simulink model "myhydro2pumps_iov1"  (Simulink 7.4)
settings: Solver=ode1  StartTime=0.0  StopTime=inf  FixedStep=0.5  RelTol=1e-3  AbsTol=1e-6
undefined symbols (not defined in the file or in its folder): calibParams, Q1max
libraries: hydro2pumps_lib x1
settings Model: Creator=dmedonza  LastModifiedBy=student
settings DataIOCC: LimitDataPoints=off  SignalLoggingName=sigsOut
settings OptimizationCC: BooleanDataType=off
settings DebuggingCC: SaveWithParameterizedLinksMsg=none  SignalResolutionControl=TryResolveAllWithWarning  SolverPrmCheckMsg=none  MultiTaskDSMMsg=warning  MultiTaskCondExecSysMsg=none  StrictBusMsg=None
settings HardwareCC: TargetUnknown=on
settings RTWCC: TemplateMakefile=grt_vc.tmf  IncludeERTFirstTime=on

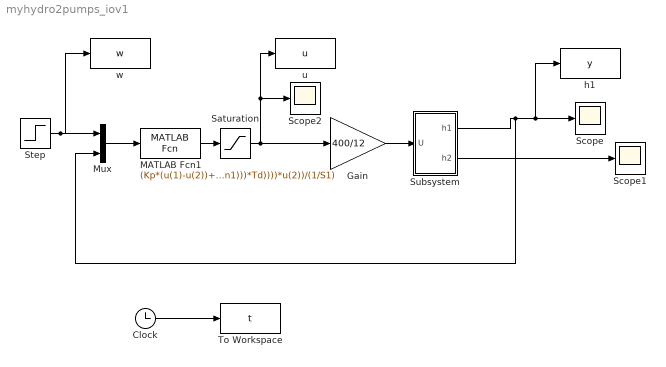
== system myhydro2pumps_iov1 ==
  Clock : Clock
      settings: Decimation=10
  Gain : Gain  Gain=400/12  ParameterDataType=fixdt(1, 16)  ParameterScaling=2^0  OutDataType=fixdt(1, 16)  OutScaling=2^0
  MATLAB Fcn1 : MATLABFcn  MATLABFcn=(Kp*(u(1)-u(2))+((1+(c1/(2*sqrt(u(2)+posun1)))*Td*exp(1+(c1/(2*sqrt(u(2)+posun1)))*Td)-exp((c1/(2*sqrt(u(2)+posun1)))*Td))/((c1/(2*sqrt(u(2)+posun1)))*Td*exp(1+(c1/(2*sqrt(u(2)+posun1)))*Td)))*u(1)+(1-((1+(c1/(2*sqrt(u(2)+posun1)))*Td*exp(1+(c1/(2*sqrt(u(2)+posun1)))*Td)-exp((c1/(2*sqrt(u(2)+posun1)))*Td))/((c1/(2*sqrt(u(2)+posun1)))*Td*exp(1+(c1/(2*sqrt(u(2)+posun1)))*Td))))*u(2))/(1/S1)
  Mux : Mux  Inputs=2
  Saturation : Saturate  UpperLimit=Q1max  LowerLimit=0  OutDataType=fixdt(1, 16)  OutScaling=2^0
  Scope : Scope
  Scope1 : Scope
  Scope2 : Scope
      settings: SaveName=ScopeData2
  Step : Step  Before=0.1  SampleTime=0
  Subsystem : Subsystem
  To Workspace : ToWorkspace  VariableName=t  SampleTime=-1  SaveFormat=Array
  h1 : ToWorkspace  VariableName=y  SampleTime=-1  SaveFormat=Array
  u : ToWorkspace  VariableName=u  SampleTime=-1  SaveFormat=Array
  w : ToWorkspace  VariableName=w  SampleTime=-1  SaveFormat=Array
  wires:
  Clock/1 -> To Workspace/1
  MATLAB Fcn1/1 -> Saturation/1
  Step/1 -> w/1, Mux/1
  Subsystem/1(h1) -> Scope/1, h1/1, Mux/2
  Subsystem/2(h2) -> Scope1/1
  Mux/1 -> MATLAB Fcn1/1
  Saturation/1 -> u/1, Scope2/1, Gain/1
  Gain/1 -> Subsystem/1(U)

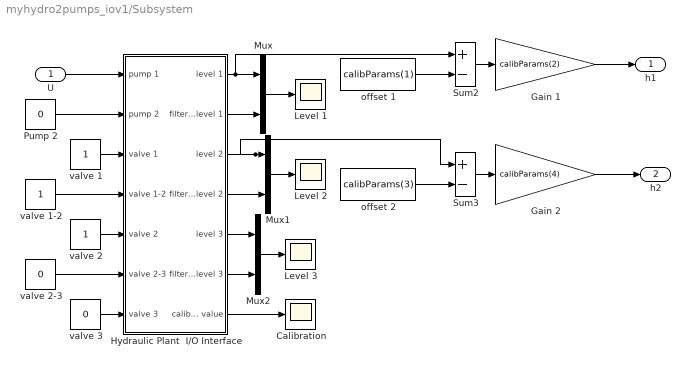
== system myhydro2pumps_iov1/Subsystem ==
  U : Inport  OutDataType=sfix(16)  OutScaling=2^0
  Calibration : Scope
      settings: TickLabels=on  TimeRange=20  YMin=0  YMax=100  SaveName=l3  DataFormat=Array
  Gain 1 : Gain  Gain=calibParams(2)  ParameterDataType=sfix(16)  ParameterScaling=2^0  OutDataType=sfix(16)  OutScaling=2^0  SaturateOnIntegerOverflow=on  OutDataTypeStr=Inherit: Same as input  ParamDataTypeStr=Inherit: Same as input
  Gain 2 : Gain  Gain=calibParams(4)  ParameterDataType=sfix(16)  ParameterScaling=2^0  OutDataType=sfix(16)  OutScaling=2^0  SaturateOnIntegerOverflow=on  OutDataTypeStr=Inherit: Same as input  ParamDataTypeStr=Inherit: Same as input
  Hydraulic Plant  I/O Interface : Subsystem
      mask Display: disp('Two Pumps\nHydraulic\nPlant\nI/O Interface')
  Level 1 : Scope
      settings: TickLabels=on  TimeRange=20  YMin=0  YMax=100  SaveName=l1  DataFormat=Array
  Level 2 : Scope
      settings: TickLabels=on  TimeRange=20  YMin=0  YMax=100  SaveName=l2  DataFormat=Array
  Level 3 : Scope
      settings: TickLabels=on  TimeRange=20  YMin=0  YMax=100  SaveName=lx  DataFormat=Array
  Mux : Mux  Inputs=2
  Mux1 : Mux  Inputs=2
  Mux2 : Mux  Inputs=2
  Pump 2 : Constant  Value=0  OutDataType=sfix(16)  OutScaling=2^0
  Sum2 : Sum  Inputs=+-  OutDataType=sfix(16)  OutScaling=2^0  SaturateOnIntegerOverflow=on
  Sum3 : Sum  Inputs=+-  OutDataType=sfix(16)  OutScaling=2^0  SaturateOnIntegerOverflow=on
  offset 1 : Constant  Value=calibParams(1)  OutDataType=sfix(16)  OutScaling=2^0
  offset 2 : Constant  Value=calibParams(3)  OutDataType=sfix(16)  OutScaling=2^0
  "valve 1 " : Constant  OutDataType=sfix(16)  OutScaling=2^0
  valve 1-2 : Constant  OutDataType=sfix(16)  OutScaling=2^0
  valve 2 : Constant  OutDataType=sfix(16)  OutScaling=2^0
  valve 2-3 : Constant  Value=0  OutDataType=sfix(16)  OutScaling=2^0
  valve 3 : Constant  Value=0  OutDataType=sfix(16)  OutScaling=2^0
  h1 : Outport
  h2 : Outport  Port=2
  wires:
  Gain 2/1 -> h2/1
  Sum3/1 -> Gain 2/1
  offset 2/1 -> Sum3/2
  Gain 1/1 -> h1/1
  Sum2/1 -> Gain 1/1
  offset 1/1 -> Sum2/2
  Mux1/1 -> Level 2/1
  Hydraulic Plant  I/O Interface/7(calibration value) -> Calibration/1
  Hydraulic Plant  I/O Interface/6(filtered level 3) -> Mux2/2
  Hydraulic Plant  I/O Interface/5(level 3) -> Mux2/1
  Hydraulic Plant  I/O Interface/4(filtered level 2) -> Mux1/2
  Hydraulic Plant  I/O Interface/3(level 2) -> Mux1/1, Sum3/1
  Hydraulic Plant  I/O Interface/2(filtered level 1) -> Mux/2
  Hydraulic Plant  I/O Interface/1(level 1) -> Mux/1, Sum2/1
  valve 3/1 -> Hydraulic Plant  I/O Interface/7(valve 3)
  valve 2-3/1 -> Hydraulic Plant  I/O Interface/6(valve 2-3)
  valve 2/1 -> Hydraulic Plant  I/O Interface/5(valve 2)
  valve 1-2/1 -> Hydraulic Plant  I/O Interface/4(valve 1-2)
  "valve 1 "/1 -> Hydraulic Plant  I/O Interface/3(valve 1)
  Pump 2/1 -> Hydraulic Plant  I/O Interface/2(pump 2)
  U/1 -> Hydraulic Plant  I/O Interface/1(pump 1)
  Mux2/1 -> Level 3/1
  Mux/1 -> Level 1/1

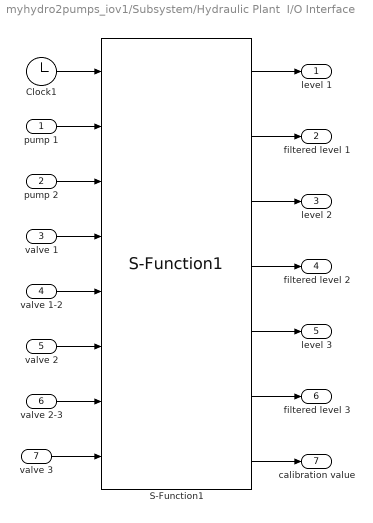
== system myhydro2pumps_iov1/Subsystem/Hydraulic Plant  I/O Interface ==
  pump 1 : Inport  OutDataType=sfix(16)  OutScaling=2^0
  pump 2 : Inport  Port=2  OutDataType=sfix(16)  OutScaling=2^0
  valve 1 : Inport  Port=3  OutDataType=sfix(16)  OutScaling=2^0
  valve 1-2 : Inport  Port=4  OutDataType=sfix(16)  OutScaling=2^0
  valve 2 : Inport  Port=5  OutDataType=sfix(16)  OutScaling=2^0
  valve 2-3 : Inport  Port=6  OutDataType=sfix(16)  OutScaling=2^0
  valve 3 : Inport  Port=7  OutDataType=sfix(16)  OutScaling=2^0
  Clock1 : Clock
      settings: Decimation=10
  S-Function1 : hydro2pumps_lib/S-Function1  Priority=1  com_port=COM4  Ts=0.5  events_ot=2  rd_timeout=250  matlab_prior=ABOVE_NORMAL_PRIORITY  warning=on  printout=off
  level 1 : Outport
  filtered level 1 : Outport  Port=2
  level 2 : Outport  Port=3
  filtered level 2 : Outport  Port=4
  level 3 : Outport  Port=5
  filtered level 3 : Outport  Port=6
  calibration value : Outport  Port=7
  wires:
  S-Function1/1 -> level 1/1
  S-Function1/2 -> filtered level 1/1
  Clock1/1 -> S-Function1/1
  pump 1/1 -> S-Function1/2
  pump 2/1 -> S-Function1/3
  S-Function1/3 -> level 2/1
  S-Function1/4 -> filtered level 2/1
  S-Function1/5 -> level 3/1
  S-Function1/6 -> filtered level 3/1
  valve 1/1 -> S-Function1/4
  valve 1-2/1 -> S-Function1/5
  valve 2/1 -> S-Function1/6
  valve 2-3/1 -> S-Function1/7
  S-Function1/7 -> calibration value/1
  valve 3/1 -> S-Function1/8
